simulink model "kers_charge_22_6_update"  (R2020a)
settings: Solver=VariableStepAuto  StartTime=0.0  StopTime=1  RelTol=1e-3
values from neighbouring files (symbols this model uses):
  d = 0.5*rho*Cx*Sf    (= 0.81)    [Data.m]
  Fn_max = 10000    [Data.m]
  Jeq_v = M*Rw^2    (= 83.853)    [Data.m]
  Jf = 1/2*(Rf^2*Mf)    (= 0.025)    [Data.m]
  k = 4/3*mi_d*R_clutch    (= 0.096)    [Data.m]
  Rw = 0.33    [Data.m]
  tau_max = 2.5    [Data.m]
  tau_min = 0.4    [Data.m]
  tau_trasm_charge = 1/(tauk_charge*tauf)    (= 52.56)    [Data.m]
  tauf = 1/4.38    (= 0.228310502283)    [Data.m]
  tauk_charge = 1/12    (= 0.0833333333333)    [Data.m]
  Tmax2 = -2457    [Data.m]
  wf_max = 64500/9.55    (= 6753.92670157)    [Data.m]
undefined symbols (not defined in the file or in its folder): tau_trasm
libraries: simulink x1
settings Model: Creator=andre  LastModifiedBy=andre
settings SFSimCC: CustomCodeUndefinedFunction=UseInterfaceOnly

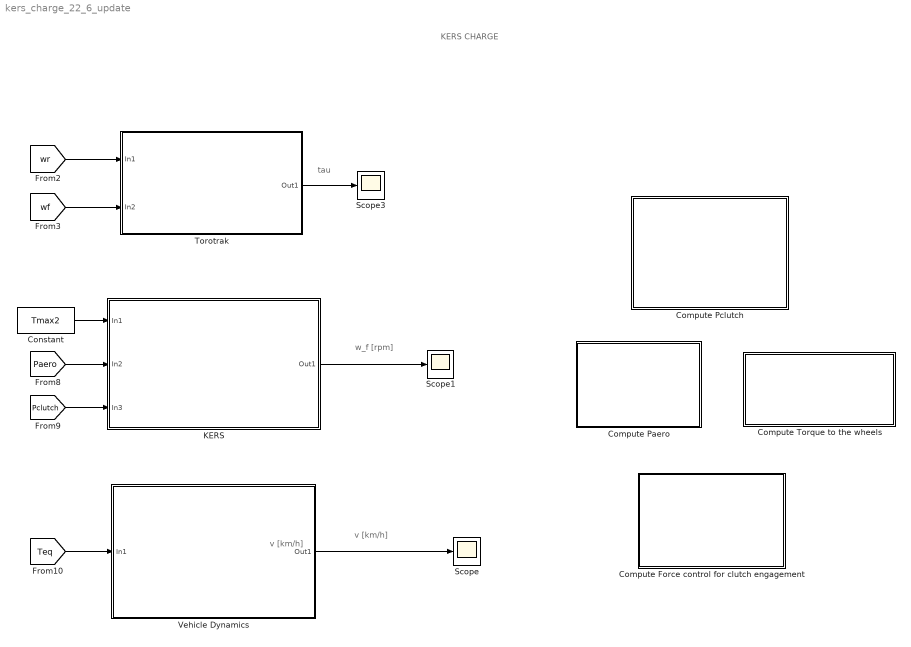
== system kers_charge_22_6_update ==
  note: KERS CHARGE
  note: v [km/h]
  note: w_f [rpm]
  note: v [km/h]
  note: tau
  Compute Force control for clutch engagement : Subsystem
  Compute Paero : Subsystem
  Compute Pclutch : Subsystem
  Compute Torque to the wheels : Subsystem
  Constant : Constant  Value=Tmax2  SampleTime=-1
  KERS : Subsystem
      mask Display: image('KERS.jpg'); % Use "Edit Image" on toolstrip to change.
  Scope : Scope
  Scope1 : Scope
  Scope3 : Scope
  Torotrak : Subsystem
      mask Display: image('Torotrak.jpg'); % Use "Edit Image" on toolstrip to change.
  Vehicle Dynamics : Subsystem
      mask Display: image('Ferrari.jpg'); % Use "Edit Image" on toolstrip to change.
  wires:
  [wr] -> Torotrak/1(In1)
  [wf] -> Torotrak/2(In2)
  Torotrak/1(Out1) -> Scope3/1
  [Teq] -> Vehicle Dynamics/1(In1)
  [Paero] -> KERS/2(In2)
  [Pclutch] -> KERS/3(In3)
  KERS/1(Out1) -> Scope1/1
  Vehicle Dynamics/1(Out1) -> Scope/1
  Constant/1 -> KERS/1(In1)

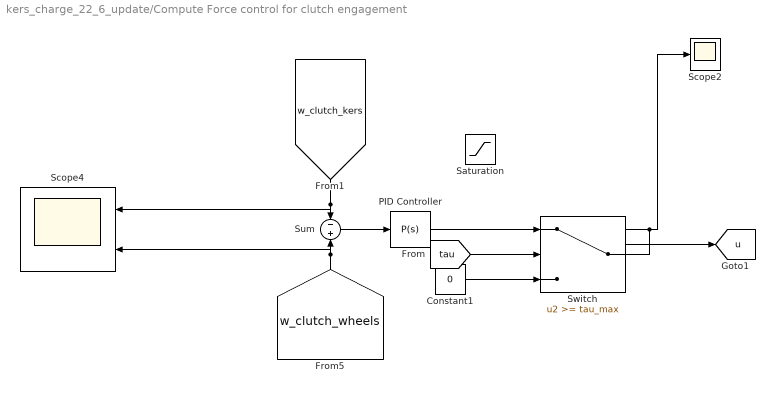
== system kers_charge_22_6_update/Compute Force control for clutch engagement ==
  Constant1 : Constant  Value=0  SampleTime=-1
  PID Controller : simulink/Continuous/PID Controller  Controller=P  Form=Parallel  TimeDomain=Continuous-time  UseExternalTs=off  SampleTime=-1  IntegratorMethod=Forward Euler  FilterMethod=Forward Euler  ControllerParametersSource=internal  P=50  I=1  D=4  UseFilter=on  N=100  TunerSelectOption=Transfer Function Based (PID Tuner App)  InitialConditionSource=internal  InitialConditionForIntegrator=0  InitialConditionForFilter=0  DifferentiatorICPrevScaledInput=0  ExternalReset=none  TrackingMode=off  Kt=1  LimitOutput=off  UpperSaturationLimit=inf  LowerSaturationLimit=-inf  LinearizeAsGain=on  AntiWindupMode=none  Kb=1  POutMin=[]  POutMax=[]  IOutMin=[]  IOutMax=[]  DOutMin=[]  DOutMax=[]  NOutMin=[]  NOutMax=[]  SumOutMin=[]  SumOutMax=[]  SaturationOutMin=[]  SaturationOutMax=[]  PParamMin=[]  PParamMax=[]  IParamMin=[]  IParamMax=[]  DParamMin=[]  DParamMax=[]  NParamMin=[]  NParamMax=[]  KbParamMin=[]  KbParamMax=[]  KtParamMin=[]  KtParamMax=[]  KbOutMin=[]  KbOutMax=[]  KtOutMin=[]  KtOutMax=[]  IntegratorOutMin=[]  IntegratorOutMax=[]  FilterOutMin=[]  FilterOutMax=[]  SumI1OutMin=[]  SumI1OutMax=[]  SumI2OutMin=[]  SumI2OutMax=[]  SumI3OutMin=[]  SumI3OutMax=[]  SumI4OutMin=[]  SumI4OutMax=[]  SumDOutMin=[]  SumDOutMax=[]  DifferentiatorOutMin=[]  DifferentiatorOutMax=[]  FilterDiffOutCoefMin=[]  FilterDiffOutCoefMax=[]  ReciprocalOutMin=[]  ReciprocalOutMax=[]  SumDenOutMin=[]  SumDenOutMax=[]  SumNumOutMin=[]  SumNumOutMax=[]  DivideOutMin=[]  DivideOutMax=[]  UdiffTsProdOutMin=[]  UdiffTsProdOutMax=[]  NTsProdOutMin=[]  NTsProdOutMax=[]  UintegralTsProdOutMin=[]  UintegralTsProdOutMax=[]  UngainTsProdOutMin=[]  UngainTsProdOutMax=[]  IntegratorContinuousStateAttributes=''  IntegratorStateMustResolveToSignalObject=off  IntegratorRTWStateStorageClass=Auto  FilterContinuousStateAttributes=''  FilterStateMustResolveToSignalObject=off  FilterRTWStateStorageClass=Auto  ParallelPVariant=InternalParameters  IdealPVariant=Disabled  IVariant=Disabled  DVariant=Disabled  IntegratorVariant=Disabled  SatVariant=Disabled  AWVariant=Disabled  PCopyVariant=Disabled  TRVariant=Disabled  FdbkBlocksVariant=Forward  IdealPFdbkVariant=Disabled  SatFdbkVariant=Disabled  DerivativeFilterVariant=Disabled  NVariant=Disabled  NCopyVariant=Disabled_SignalSpec  FilterICVariant=Disabled  IntegratorICVariant=Disabled  ExternalResetVariant=Disabled  TRSumVariant=Passthrough  SumFdbkVariant=Disabled  SumVariant=Passthrough_P  TsampFilterVariant=InternalTs  TsampNgainVariant=Passthrough  TsampIntegralVariant=Disabled_SignalSpec
  Saturation : Saturate  UpperLimit=Fn_max  LowerLimit=-Fn_max
  Scope2 : Scope
  Scope4 : Scope  NumInputPorts=2
  Sum : Sum  Inputs=-+
  Switch : Switch  Threshold=tau_max
  tag scope: u=global
  wires:
  Switch/1 -> [u], Scope2/1
  Sum/1 -> PID Controller/1
  Constant1/1 -> Switch/3
  [tau] -> Switch/2
  [w_clutch_kers] -> Scope4/1, Sum/1
  [w_clutch_wheels] -> Scope4/2, Sum/2
  PID Controller/1 -> Switch/1

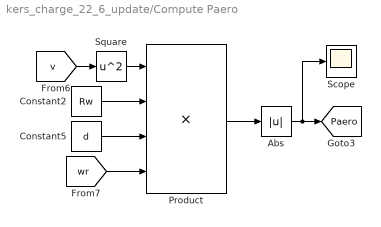
== system kers_charge_22_6_update/Compute Paero ==
  Abs : Abs  ZeroCross=off
  Constant2 : Constant  Value=Rw
  Constant5 : Constant  Value=d
  Product : Product  Inputs=4
  Scope : Scope
  Square : Math  Operator=square  SignedPower=on  SaturateOnIntegerOverflow=on
  tag scope: Paero=global
  wires:
  Square/1 -> Product/1
  Constant5/1 -> Product/3
  [wr] -> Product/4
  [v] -> Square/1
  Constant2/1 -> Product/2
  Product/1 -> Abs/1
  Abs/1 -> Scope/1, [Paero]

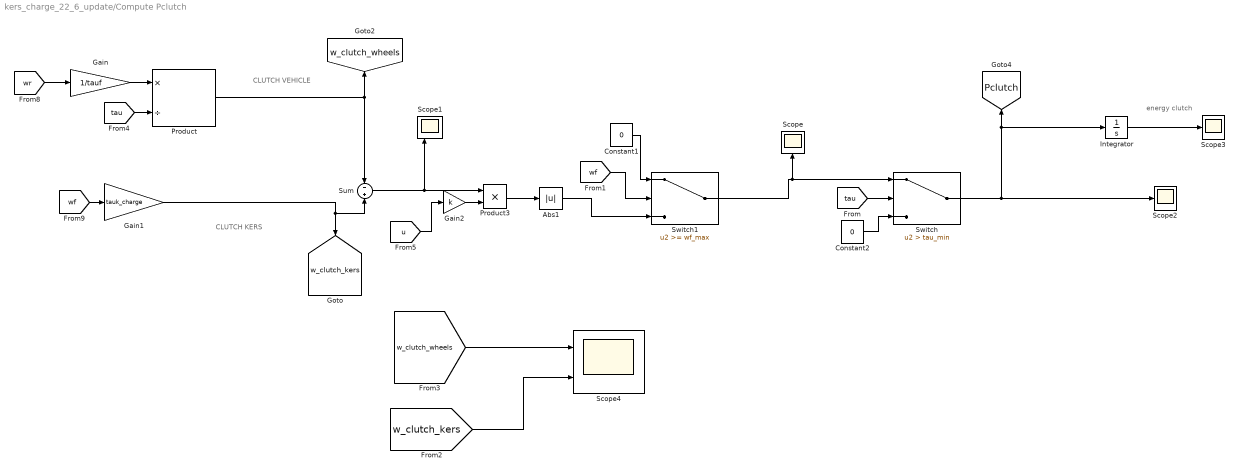
== system kers_charge_22_6_update/Compute Pclutch ==
  note: CLUTCH KERS
  note: CLUTCH VEHICLE
  note: energy clutch
  Abs1 : Abs  ZeroCross=off
  Constant1 : Constant  Value=0
  Constant2 : Constant  Value=0
  Gain : Gain  Gain=1/tauf
  Gain1 : Gain  Gain=tauk_charge
  Gain2 : Gain  Gain=k
  Integrator : Integrator
  Product : Product  Inputs=*/
  Product3 : Product
  Scope : Scope
  Scope1 : Scope  NumInputPorts=2
  Scope2 : Scope
  Scope3 : Scope
  Scope4 : Scope  NumInputPorts=2
  Sum : Sum  Inputs=-+
  Switch : Switch  Criteria=u2 > Threshold  Threshold=tau_min
  Switch1 : Switch  Threshold=wf_max
  tag scope: Pclutch=global, w_clutch_kers=global, w_clutch_wheels=global
  wires:
  Gain1/1 -> [w_clutch_kers], Sum/2
  Sum/1 -> Product3/1, Scope1/1
  Product3/1 -> Abs1/1
  Integrator/1 -> Scope3/1
  [wf] -> Switch1/2
  Constant1/1 -> Switch1/1
  Abs1/1 -> Switch1/3
  [tau] -> Switch/2
  Switch1/1 -> Switch/1, Scope/1
  Constant2/1 -> Switch/3
  Switch/1 -> Integrator/1, [Pclutch], Scope2/1
  [wr] -> Gain/1
  Gain/1 -> Product/1
  [tau] -> Product/2
  Product/1 -> [w_clutch_wheels], Sum/1
  [wf] -> Gain1/1
  [w_clutch_kers] -> Scope4/2
  [w_clutch_wheels] -> Scope4/1
  [u] -> Gain2/1
  Gain2/1 -> Product3/2

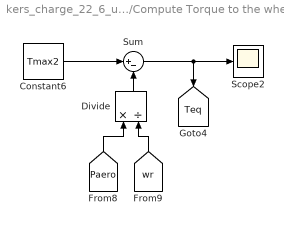
== system kers_charge_22_6_update/Compute Torque to the wheels ==
  Constant6 : Constant  Value=Tmax2
  Divide : Product  Inputs=*/
  Scope2 : Scope
  Sum : Sum  Inputs=|+-
  tag scope: Teq=global
  wires:
  Sum/1 -> [Teq], Scope2/1
  [Paero] -> Divide/1
  Constant6/1 -> Sum/1
  [wr] -> Divide/2
  Divide/1 -> Sum/2

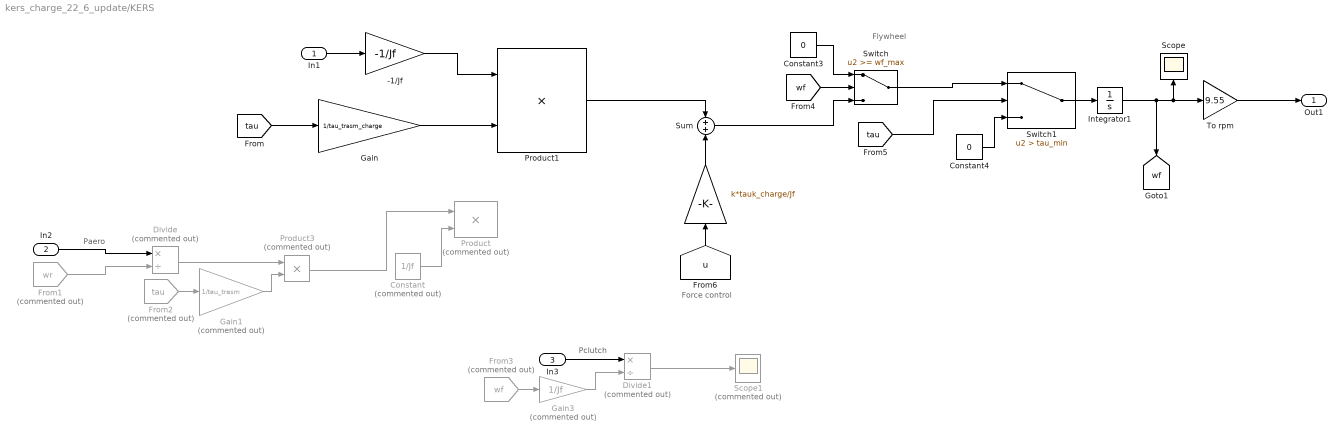
== system kers_charge_22_6_update/KERS ==
  note: Force control
  note: Pclutch
  note: Paero
  note: Flywheel
  In1 : Inport
  In2 : Inport  Port=2
  In3 : Inport  Port=3
  " " : Gain  Gain=k*tauk_charge/Jf
  -1/Jf : Gain  Gain=-1/Jf
  Constant : Constant  Commented=on  Value=1/Jf
  Constant3 : Constant  Value=0
  Constant4 : Constant  Value=0
  Divide : Product  Commented=on  Inputs=*/
  Divide1 : Product  Commented=on  Inputs=*/
  From1 : From  Commented=on  GotoTag=wr  TagVisibility=global
  From2 : From  Commented=on  GotoTag=tau  TagVisibility=global
  From3 : From  Commented=on  GotoTag=wf  TagVisibility=global
  Gain : Gain  Gain=1/tau_trasm_charge
  Gain1 : Gain  Commented=on  Gain=1/tau_trasm
  Gain3 : Gain  Commented=on  Gain=1/Jf
  Integrator1 : Integrator  InitialCondition=0.0001  ContinuousStateAttributes="\"omega_f\""
  Product : Product  Commented=on  Inputs=**
  Product1 : Product  Inputs=**
  Product3 : Product  Commented=on
  Scope : Scope
  Scope1 : Scope  Commented=on
  Sum : Sum
  Switch : Switch  Threshold=wf_max
  Switch1 : Switch  Criteria=u2 > Threshold  Threshold=tau_min
  To rpm : Gain  Gain=9.55
  Out1 : Outport
  tag scope: wf=global
  wires:
  Sum/1 -> Switch/3
  Switch1/1 -> Integrator1/1
  -1/Jf/1 -> Product1/1
  Integrator1/1 -> Scope/1, To rpm/1, [wf]
  Constant3/1 -> Switch/1
  Switch/1 -> Switch1/1
  [wf] -> Switch/2
  Constant4/1 -> Switch1/3
  [tau] -> Switch1/2
  Product1/1 -> Sum/1
  To rpm/1 -> Out1/1
  In1/1 -> -1/Jf/1
  Gain/1 -> Product1/2
  [tau] -> Gain/1
  In2/1 -> Divide/1
  From1/1 -> Divide/2
  Divide/1 -> Product3/1
  From2/1 -> Gain1/1
  Gain1/1 -> Product3/2
  Product3/1 -> Product/1
  Constant/1 -> Product/2
  In3/1 -> Divide1/1
  From3/1 -> Gain3/1
  Gain3/1 -> Divide1/2
  Divide1/1 -> Scope1/1
  [u] -> " "/1
  " "/1 -> Sum/2

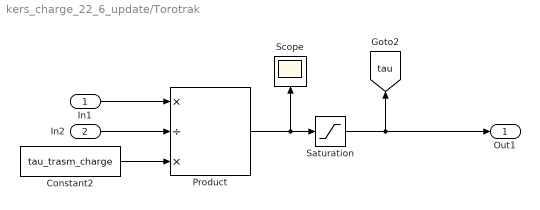
== system kers_charge_22_6_update/Torotrak ==
  In1 : Inport
  In2 : Inport  Port=2
  Constant2 : Constant  Value=tau_trasm_charge
  Product : Product  Inputs=*/*
  Saturation : Saturate  UpperLimit=tau_max  LowerLimit=tau_min
  Scope : Scope
  Out1 : Outport
  tag scope: tau=global
  wires:
  In2/1 -> Product/2
  Constant2/1 -> Product/3
  Saturation/1 -> Out1/1, [tau]
  In1/1 -> Product/1
  Product/1 -> Scope/1, Saturation/1

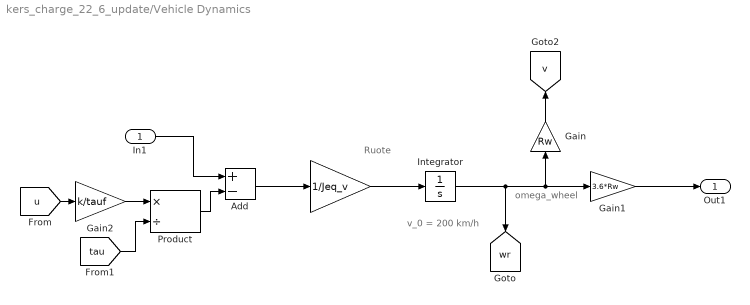
== system kers_charge_22_6_update/Vehicle Dynamics ==
  note: omega_wheel
  note: v_0 = 200 km/h
  note: Ruote
  In1 : Inport
  " " : Gain  Gain=1/Jeq_v
  Add : Sum  Inputs=+-
  Gain : Gain  Gain=Rw
  Gain1 : Gain  Gain=3.6*Rw
  Gain2 : Gain  Gain=k/tauf
  Integrator : Integrator  InitialCondition=300/(3.6*Rw)  ContinuousStateAttributes='omega_w'
  Product : Product  Inputs=*/
  Out1 : Outport
  tag scope: v=global, wr=global
  wires:
  Integrator/1 -> Gain/1, Gain1/1, [wr]
  Gain/1 -> [v]
  " "/1 -> Integrator/1
  Gain1/1 -> Out1/1
  In1/1 -> Add/1
  Add/1 -> " "/1
  [u] -> Gain2/1
  Gain2/1 -> Product/1
  [tau] -> Product/2
  Product/1 -> Add/2
